simulink model "ftm_qd_s32k14x"  (Simulink 9.0)
settings: Solver=FixedStepDiscrete  StartTime=0.0  StopTime=10.0  FixedStep=0.5  RelTol=1e-3  EnableMultiTasking=on
InitFcn:
  | mbd_s32k_consistency_checks(bdroot(gcs));
undefined symbols (not defined in the file): LQFP
libraries: mbd_s32k1xx_ec_toolbox x10, simulink x1
Description:
  | This model shows FlexTimer Quadrature Decoder Mode.
  | 
  | Connect PTA15 output to FTM1 Phase A input PTA1
  | Connect PTB4 output to FTM1 Phase B input PTB2
  | 
  | Connect PTA7 output to FTM2 Phase A input PTA0
  | Connect PTA13 output to FTM2 Phase B input PTA12
  | 
  | Validation:
  | You can see FTM1 Counter value increment and decrement
  | in Count and Direction Mode by FreeMaster.
  | 
  | You can see FTM2 CounterAB value increment and decrement
  | in PhaseA and PhaseB Encoding Mode by FreeMaster.
settings Model: Creator=NXP MBDT Team  LastModifiedBy=nxf35172
settings DataIOCC: ExternalInput=off  InitialState=off  LimitDataPoints=on  SaveOutput=off  SignalLogging=off  SaveTime=off
settings OptimizationCC: DefaultParameterBehavior=Inlined  LifeSpan=1
settings DebuggingCC: SolverPrmCheckMsg=warning  InheritedTsInSrcMsg=none  SingleTaskRateTransMsg=error  UnconnectedInputMsg=error  UnconnectedOutputMsg=error  UnconnectedLineMsg=error  AllowSymbolicDim=off  UnknownTsInhSupMsg=error  StateNameClashWarn=warning
settings HardwareCC: ProdLargestAtomicInteger=Long  ProdLargestAtomicFloat=Double  ProdEndianess=LittleEndian  ProdHWDeviceType=ARM Compatible->ARM Cortex
settings SFSimCC: MATLABDynamicMemAlloc=off
settings RTWCC: SystemTargetFile=mbd_s32k.tlc  MakeCommand=mbd_s32k_make_rtw COPY_MDLREF_INCLUDES=0  TemplateMakefile=mbd_s32k.tmf  Description=Model Based Design Toolbox S32K14x Code Generation Target  GenerateReport=on  LaunchReport=on
settings CodeAppCC: IgnoreCustomStorageClasses=off
settings STFCustomTargetCC: CombineOutputUpdateFcns=on  ERTCustomFileBanners=on  SupportContinuousTime=off  SupportNonInlinedSFcns=off  RemoveResetFunc=on  MATLABClassNameForMDSCustomization=Simulink.SoftwareTarget.ERTCustomization  GRTInterface=off  SystemTargetFile=mbd_s32k14.tlc
settings ERTTargetCC: MultiwordLength=2048  ParMdlRefBuildCompliant=off  CompOptLevelCompliant=off  ConcurrentExecutionCompliant=off  ModelStepFunctionPrototypeControlCompliant=off  CPPClassGenCompliant=off  UseToolchainInfoCompliant=off  InlinedParameterPlacement=NonHierarchical  ERTCustomFileTemplate=example_file_process.tlc  ConvertIfToSwitch=off  SuppressUnreachableDefaultCases=off

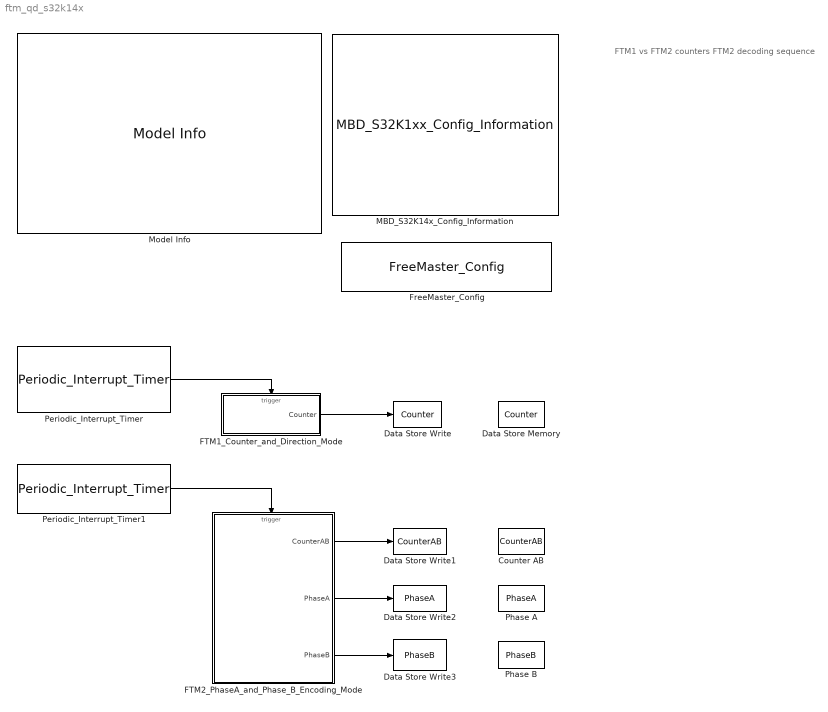
== system ftm_qd_s32k14x ==
  note: FTM1 vs FTM2 counters
      |
      | FTM2 decoding sequence
  Counter AB : DataStoreMemory  DataStoreName=CounterAB  ReadBeforeWriteMsg=warning  WriteAfterWriteMsg=warning  WriteAfterReadMsg=warning  ShowAdditionalParam=off  OutDataTypeStr=uint16
  Data Store Memory : DataStoreMemory  DataStoreName=Counter  ReadBeforeWriteMsg=warning  WriteAfterWriteMsg=warning  WriteAfterReadMsg=warning  ShowAdditionalParam=off  OutDataTypeStr=uint16
  Data Store Write : DataStoreWrite  DataStoreName=Counter
  Data Store Write1 : DataStoreWrite  DataStoreName=CounterAB
  Data Store Write2 : DataStoreWrite  DataStoreName=PhaseA
  Data Store Write3 : DataStoreWrite  DataStoreName=PhaseB
  FTM1_Counter_and_Direction_Mode : Subsystem  TreatAsAtomicUnit=on
      settings: RTWSystemCode=Nonreusable function
  FTM2_PhaseA_and_Phase_B_Encoding_Mode : Subsystem  TreatAsAtomicUnit=on
      settings: RTWSystemCode=Nonreusable function
  FreeMaster_Config : mbd_s32k1xx_ec_toolbox/Utility Blocks/FreeMaster_Config  interface=LPUART1  baudrate=115200  rxd=PTC6: [LPUART1_RX | Receive]  txd=PTC7: [LPUART1_TX | Transmit]  mode=Short Interrupt  isr_prio=0  show_adv_opts=off  use_scope=on  max_scope_vars=8  use_recorder=on  max_rec_vars=8  rec_buff_size=1024  rec_timebase=0 milliseconds  comm_buffer_size_auto=on  comm_buffer_size=255  comm_rqueue_size_default=on  comm_rqueue_size=32
  MBD_S32K14x_Config_Information : mbd_s32k1xx_ec_toolbox/MBD_S32K1xx_Config_Information  mbdt_ver=0  disp_str=|  config_params=[]  mcu_target_name=S32K144  mcu_target_package=100-LQFP  mcu_target_sram_size=64KB  mcu_system_clock_freq=80  mcu_xtal_freq=External 8  mcu_steptick_timer=LPIT Channel 0  mcu_steptick_prio=0  ds_import_enable=on  target_compiler=GCC  target_memory=FLASH  gcc_target_compile_opts=-mcpu=cortex-m4 -mthumb -mfloat-abi=hard -mfpu=fpv4-sp-d16 -O1 -g -gstrict-dwarf  gcc_target_assemble_opts=-mcpu=cortex-m4 -mthumb -mfloat-abi=hard -mfpu=fpv4-sp-d16 -g  gcc_target_link_opts=-mcpu=cortex-m4 -mthumb -mfloat-abi=hard -mfpu=fpv4-sp-d16  gcc_target_default_lcf=on  gcc_target_user_lcf=S32K144_64_flash.ld  ghs_target_compile_opts=-cpu=cortexm4f -thumb -DARM_MATH_CM4 -fpu=vfpv4_d16 -fsingle -Ogeneral -Wundef -Wimplicit-int -Wshadow -Wtrigraphs --no_commons --gnu_asm -gnu99 -gdwarf-2 -G  ghs_target_assemble_opts=-cpu=cortexm4f -fpu=vfpv4_d16  ghs_target_link_opts=-cpu=cortexm4f -thumb -fpu=vfpv4_d16  ghs_target_default_lcf=off  ghs_target_user_lcf=S32K144_64_flash.ld  iar_target_compile_opts=--cpu=Cortex-M4F --thumb --fpu=VFPv4_sp -Ol -e --debug --dlib_config normal  iar_target_assemble_opts=--cpu Cortex-M4F --thumb --fpu VFPv4_sp  iar_target_link_opts=--no_exceptions --vfe --inline  iar_target_default_lcf=off  iar_target_user_lcf=S32K144_64_flash.icf  pil_download_enable=off  rbl_download_enable=on  rbl_start_delay=5000000  rbl_download_interface=OpenSDA  rbl_restart_request=off  rbl_com_port=Custom  rbl_com_port_custom=COM1  pil_download_rate=57600  pil_opensda_drive=Custom  pil_opensda_drive_custom=D  pil_uart_instance=0  pil_uart_rx=PTA2: [LPUART0_RX | Receive]  pil_uart_tx=PTA3: [LPUART0_TX | Transmit]  FTM_PWM_PcrCheckEnDis=on  FTM_Input_Edge_Inputs_PcrCheckEnDis=on  FTM_Dual_Edge_Inputs_PcrCheckEnDis=on  FTM_Quadrature_Inputs_PcrCheckEnDis=on  FTM_Hall_Sensor_Inputs_PcrCheckEnDis=on  LPTMR_PcrCheckEnDis=on  PIT_PcrCheckEnDis=on  RTC_PcrCheckEnDis=on  FlexCAN_PcrCheckEnDis=on  LIN_PcrCheckEnDis=on  FlexIO_PcrCheckEnDis=on  LPI2C_PcrCheckEnDis=on  LPSPI_PcrCheckEnDis=on  LPUART_PcrCheckEnDis=on  CMP_PcrCheckEnDis=on  GPIO_OutputPcrCheckEnDis=on  GPIO_InputPcrCheckEnDis=on  SBC_PcrCheckEnDis=on  AMMCLIB_PcrCheckEnDis=on  FM_PcrCheckEnDis=on  Profile_PcrCheckEnDis=on  ConfigParams_PcrCheckEnDis=on  ModelRef_PcrCheckEnDis=on  PDB0_PcrCheckEnDis=on  CSEc_PcrCheckEnDis=on  eDMA_PcrCheckEnDis=on  ADC_PcrCheckEnDis=on  WDOG_PcrCheckEnDis=on
      | Target : S32K144-48KB_SRAM
      | Package : 100-pin
      | System clock : 80 MHz
      | XTAL clock : External 8 MHz
      | Compiler : IAR
      | Target Type : FLASH
      | Download Code after build : off
      | Step Tick Interrupt Priority : 15
  Model Info : simulink/Model-Wide Utilities/Model Info  Frame=off  DisplayStringWithTags=|  HorizontalTextAlignment=Left  LeftAlignmentValue=0.02
      | Model Name: %<ModelName>
      | 
      | Description: %<Description>
  Periodic_Interrupt_Timer : mbd_s32k1xx_ec_toolbox/Utility Blocks/Periodic_Interrupt_Timer  channel=2  period=10000  prio=0  startCounter=on
  Periodic_Interrupt_Timer1 : mbd_s32k1xx_ec_toolbox/Utility Blocks/Periodic_Interrupt_Timer  channel=3  period=100000  prio=0  startCounter=on
  Phase A : DataStoreMemory  DataStoreName=PhaseA  ReadBeforeWriteMsg=warning  WriteAfterWriteMsg=warning  WriteAfterReadMsg=warning  ShowAdditionalParam=off  OutDataTypeStr=boolean
  Phase B : DataStoreMemory  DataStoreName=PhaseB  ReadBeforeWriteMsg=warning  WriteAfterWriteMsg=warning  WriteAfterReadMsg=warning  ShowAdditionalParam=off  OutDataTypeStr=boolean
  wires:
  Periodic_Interrupt_Timer/1 -> FTM1_Counter_and_Direction_Mode/Trigger
  FTM1_Counter_and_Direction_Mode/1(Counter) -> Data Store Write/1
  Periodic_Interrupt_Timer1/1 -> FTM2_PhaseA_and_Phase_B_Encoding_Mode/Trigger
  FTM2_PhaseA_and_Phase_B_Encoding_Mode/1(CounterAB) -> Data Store Write1/1
  FTM2_PhaseA_and_Phase_B_Encoding_Mode/2(PhaseA) -> Data Store Write2/1
  FTM2_PhaseA_and_Phase_B_Encoding_Mode/3(PhaseB) -> Data Store Write3/1

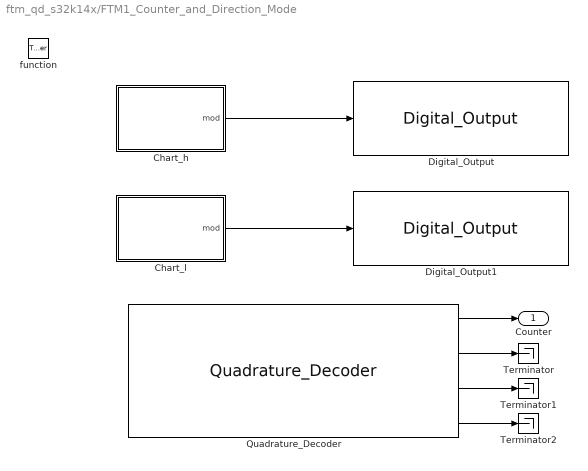
== system ftm_qd_s32k14x/FTM1_Counter_and_Direction_Mode ==
  function : TriggerPort  TriggerType=function-call  VariantControl=Variant
  Chart_h : Stateflow chart  TreatAsAtomicUnit=on
  Chart_l : Stateflow chart  TreatAsAtomicUnit=on
  Digital_Output : mbd_s32k1xx_ec_toolbox/GPIO Blocks/Digital_Output  gpio_pin=PTA15: [PTA15 | Port A I/O]  init_val=Low  drive_strength=Low
  Digital_Output1 : mbd_s32k1xx_ec_toolbox/GPIO Blocks/Digital_Output  gpio_pin=PTB4: [PTB4 | Port B I/O]  init_val=Low  drive_strength=Low
  Quadrature_Decoder : mbd_s32k1xx_ec_toolbox/Motor Control Blocks/FTM Blocks/Quadrature_Decoder  Priority=1  ftmModule=1  ec_mode=Count and Direction  prescaler=1  cntin=0  mod=65535  phA_filtr_en=off  phA_filter=0  phA_pin=PTA1: [FTM1_QD_PHA | FTM quadrature Decode PhaseA]  polA=Normal  phB_filtr_en=off  phB_filter=0  phB_pin=PTB2: [FTM1_QD_PHB | FTM quadrature Decode PhaseB]  polB=Normal
  Terminator : Terminator
  Terminator1 : Terminator
  Terminator2 : Terminator
  Counter : Outport
  wires:
  Chart_h/1(mod) -> Digital_Output/1
  Chart_l/1(mod) -> Digital_Output1/1
  Quadrature_Decoder/1 -> Counter/1
  Quadrature_Decoder/2 -> Terminator/1
  Quadrature_Decoder/4 -> Terminator2/1
  Quadrature_Decoder/3 -> Terminator1/1

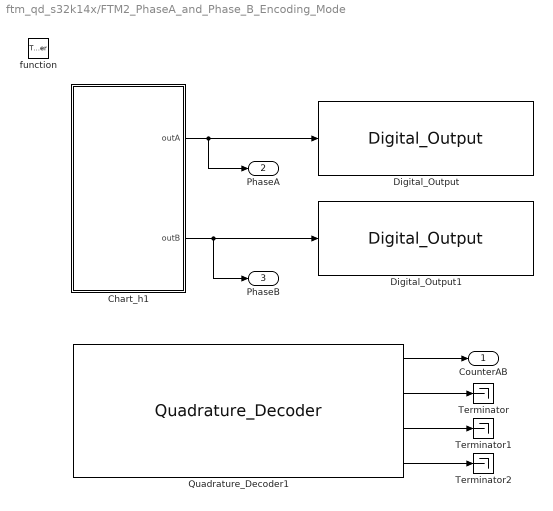
== system ftm_qd_s32k14x/FTM2_PhaseA_and_Phase_B_Encoding_Mode ==
  function : TriggerPort  TriggerType=function-call  VariantControl=Variant
  Chart_h1 : Stateflow chart  TreatAsAtomicUnit=on
  Digital_Output : mbd_s32k1xx_ec_toolbox/GPIO Blocks/Digital_Output  gpio_pin=PTA7: [PTA7 | Port A I/O]  init_val=Low  drive_strength=Low
  Digital_Output1 : mbd_s32k1xx_ec_toolbox/GPIO Blocks/Digital_Output  gpio_pin=PTA13: [PTA13 | Port A I/O]  init_val=Low  drive_strength=Low
  Quadrature_Decoder1 : mbd_s32k1xx_ec_toolbox/Motor Control Blocks/FTM Blocks/Quadrature_Decoder  Priority=1  ftmModule=2  ec_mode=Phase A and Phase B  prescaler=1  cntin=0  mod=65535  phA_filtr_en=off  phA_filter=0  phA_pin=PTA0: [FTM2_QD_PHA | FTM quadrature Decode PhaseA]  polA=Normal  phB_filtr_en=off  phB_filter=0  phB_pin=PTA12: [FTM2_QD_PHB | FTM quadrature Decode PhaseB]  polB=Normal
  Terminator : Terminator
  Terminator1 : Terminator
  Terminator2 : Terminator
  CounterAB : Outport
  PhaseA : Outport  Port=2
  PhaseB : Outport  Port=3
  wires:
  Quadrature_Decoder1/1 -> CounterAB/1
  Chart_h1/1(outA) -> Digital_Output/1, PhaseA/1
  Chart_h1/2(outB) -> Digital_Output1/1, PhaseB/1
  Quadrature_Decoder1/2 -> Terminator/1
  Quadrature_Decoder1/3 -> Terminator1/1
  Quadrature_Decoder1/4 -> Terminator2/1

== stateflow chart FTM1_Counter_and_Direction_Mode/Chart_h ==
  state A
    du:
    mod = 0;
    cntr=cntr+1;
  state A1
    du:
    mod = 1;
    cntr=cntr+1;
  (default) -> A : {cntr = 1;}
  A1 -> A : [cntr==4]
      | {cntr=0;}
  A -> A1 : [cntr == 4]
      | {cntr = 0;}
  data: cntr local uint16; mod output boolean

== stateflow chart FTM1_Counter_and_Direction_Mode/Chart_l ==
  state A
    du:
    mod = 1;
    cntr=cntr+1;
  state A1
    du:
    mod = 0;
    cntr=cntr+1;
  (default) -> A : {cntr = -10;}
  A1 -> A : [cntr==999]
      | {cntr=0;}
  A -> A1 : [cntr == 999]
      | {cntr = 0;}
  data: cntr local int16; mod output boolean

== stateflow chart FTM2_PhaseA_and_Phase_B_Encoding_Mode/Chart_h1 ==
  state A0
    du:
    cntr=cntr+1;
  state A1
    du:
    cntr=cntr+1;
  state A2
    du:
    cntr=cntr+1;
  state A3
    du:
    cntr=cntr+1;
  state A4
    du:
    cntr=cntr+1;
  state A5
    du:
    cntr=cntr+1;
  A4 -> A5 : [cntr == 9]
      | {cntr = 0; outB = ~outB;}
  A3 -> A4 [order 2] : [(cntr == 9)&&(rep == 5)]
      | {cntr = 0; rep = 0;}
  A5 -> A0 : [cntr == 9]
      | {cntr = 0; outA = 1;}
  (default) -> A0 : {cntr = 0; rep = 0;
      | outA=1; outB = 0;}
  A3 -> A0 [order 1] : [(cntr == 9)&&(rep < 5)]
      | {cntr = 0; outA = 1;}
  A2 -> A3 : [cntr == 9]
      | {cntr = 0; rep = rep + 1;
      | outB = ~outB;}
  A0 -> A1 : [cntr == 9]
      | {cntr = 0;
      | outB = ~outB;}
  A1 -> A2 : [cntr == 9]
      | {cntr = 0; outA = 0;}
  data: cntr local uint16; outA output boolean; rep local uint16; outB output boolean
